simulink library "ADV_IP_MASTER"  (Simulink 8.6)
settings: Solver=VariableStepAuto  StartTime=0.0  StopTime=10.0  RelTol=1e-3
libraries: cdsEpicsOut x45, cdsFiltCtrl x25, cdsFilt x19, cdsEpicsIn x16, cdsTP x6, cdsMuxMatrix x4, VIS_LIB x1, cdsRampMuxMatrix x1, cdsFunctionCall x1, SIXOSEM_F_WD_AC_MASTER x1, SIXOSEM_F_STAGE_MASTER x1
(part 3 of 5)

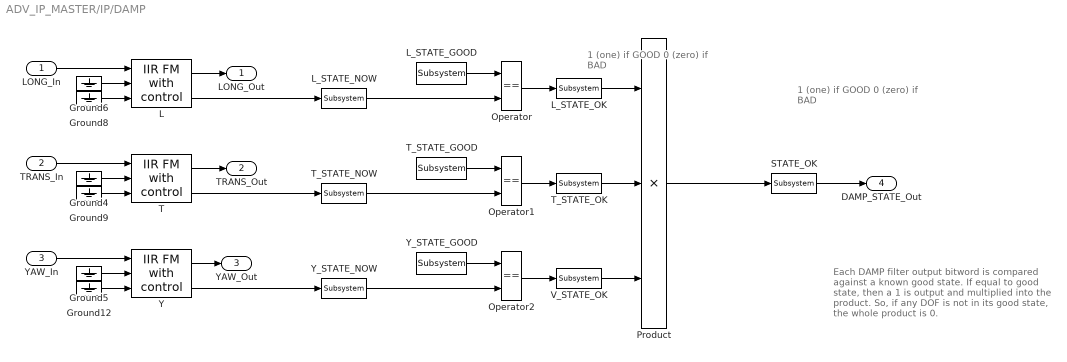
== system ADV_IP_MASTER/IP/DAMP ==
  note: 1 (one) if GOOD
      | 0 (zero) if BAD
  note: 1 (one) if GOOD
      | 0 (zero) if BAD
  note: Each DAMP filter output bitword is
      | compared against a known good state.
      | If equal to good state, then a 1 is output
      | and multiplied into the product. So, if any DOF
      | is not in its good state, the whole product is 0.
  LONG_In : Inport
  TRANS_In : Inport  Port=2
  YAW_In : Inport  Port=3
  Ground{4..6,8..9,12} (6 alike) : Ground
  L : cdsFiltCtrl/IIR FM with control  Tag=cdsFiltCtrl  Description=|
      | cdsFiltCntrl is the standard IIR filter module (exactly the same as cdsFilt) but with added control data output 'Ctrl'. Filter module digital signal output appears on the first output, which is called 'Val'. 'Ctrl' output has a bit pattern encoding the state of filter's on/off switches (FM1 through FM10). The bit values are:
      |                                                                                                                                                                                                                                                                                                                                       
      | module 	hex	dec                                                                                                                                                                                                                                                                                                                       
      | -----------------------                                                                                                                                                                                                                                                                                                               
      | FM1	0x20                    32                                                                                                                                                                                                                                                                                                        
      | FM2	0x80                     128                                                                                                                                                                                                                                                                                                      
      | FM3	0x200                   512                                                                                                                                                                                                                                                                                                       
      | FM4	0x800                   2048                                                                                                                                                                                                                                                                                                      
      | FM5	0x2000                 8192                                                                                                                                                                                                                                                                                                       
      | FM6	0x8000                 32768                                                                                                                                                                                                                                                                                                      
      | FM7	0x20000                131072                                                                                                                                                                                                                                                                                                     
      | FM8	0x80000                 524288                                                                                                                                                                                                                                                                                                    
      | FM9	0x200000               2097152                                                                                                                                                                                                                                                                                                    
      | FM10	0x800000               8388608                                                                                                                                                                                                                                                                                                   
      |                                                                                                                                                                                                                                                                                                                                       
      | This bit data can be used to drive some other switches or it can be output using a binary I/O module.
      settings: AttributesFormatString=%<Tag>
  L_STATE_GOOD : cdsEpicsIn/Subsystem  Tag=cdsEpicsIn  Description=|
      | Purpose:                                                                              
      | Create an EPICS input channel connection to the FE realtime controls.                 
      |                                                                                       
      | Operation:                                                                            
      | Outputs value from an EPICS ai record. Value is floating point with a precision of 3..
      |                                                                                       
      | Usage:                                                                                
      | Name the part with the desired EPICS channel name.
      settings: AttributesFormatString=%<Tag>
  L_STATE_NOW : cdsEpicsOut/Subsystem  Tag=cdsEpicsOutput  Description=|
      | Purpose:                                          
      | Output a FE signal to an EPICS channel.           
      |                                                   
      | Operation:                                        
      | Takes input value and passes it to EPICS record.  
      |                                                   
      | Usage:                                            
      | Name the part with the desired EPICS rrecord name.
      settings: AttributesFormatString=%<Tag>
  L_STATE_OK : cdsEpicsOut/Subsystem  Tag=cdsEpicsOutput  Description=|
      | Purpose:                                          
      | Output a FE signal to an EPICS channel.           
      |                                                   
      | Operation:                                        
      | Takes input value and passes it to EPICS record.  
      |                                                   
      | Usage:                                            
      | Name the part with the desired EPICS rrecord name.
      settings: AttributesFormatString=%<Tag>
  Operator : RelationalOperator  Operator===  OutDataTypeStr=boolean
  Operator1 : RelationalOperator  Operator===  OutDataTypeStr=boolean
  Operator2 : RelationalOperator  Operator===  OutDataTypeStr=boolean
  Product : Product  Inputs=3  RndMeth=Zero
  STATE_OK : cdsEpicsOut/Subsystem  Tag=cdsEpicsOutput  Description=|
      | Purpose:                                          
      | Output a FE signal to an EPICS channel.           
      |                                                   
      | Operation:                                        
      | Takes input value and passes it to EPICS record.  
      |                                                   
      | Usage:                                            
      | Name the part with the desired EPICS rrecord name.
      settings: AttributesFormatString=%<Tag>
  T : cdsFiltCtrl/IIR FM with control  Tag=cdsFiltCtrl  Description=|
      | cdsFiltCntrl is the standard IIR filter module (exactly the same as cdsFilt) but with added control data output 'Ctrl'. Filter module digital signal output appears on the first output, which is called 'Val'. 'Ctrl' output has a bit pattern encoding the state of filter's on/off switches (FM1 through FM10). The bit values are:
      |                                                                                                                                                                                                                                                                                                                                       
      | module 	hex	dec                                                                                                                                                                                                                                                                                                                       
      | -----------------------                                                                                                                                                                                                                                                                                                               
      | FM1	0x20                    32                                                                                                                                                                                                                                                                                                        
      | FM2	0x80                     128                                                                                                                                                                                                                                                                                                      
      | FM3	0x200                   512                                                                                                                                                                                                                                                                                                       
      | FM4	0x800                   2048                                                                                                                                                                                                                                                                                                      
      | FM5	0x2000                 8192                                                                                                                                                                                                                                                                                                       
      | FM6	0x8000                 32768                                                                                                                                                                                                                                                                                                      
      | FM7	0x20000                131072                                                                                                                                                                                                                                                                                                     
      | FM8	0x80000                 524288                                                                                                                                                                                                                                                                                                    
      | FM9	0x200000               2097152                                                                                                                                                                                                                                                                                                    
      | FM10	0x800000               8388608                                                                                                                                                                                                                                                                                                   
      |                                                                                                                                                                                                                                                                                                                                       
      | This bit data can be used to drive some other switches or it can be output using a binary I/O module.
      settings: AttributesFormatString=%<Tag>
  T_STATE_GOOD : cdsEpicsIn/Subsystem  Tag=cdsEpicsIn  Description=|
      | Purpose:                                                                              
      | Create an EPICS input channel connection to the FE realtime controls.                 
      |                                                                                       
      | Operation:                                                                            
      | Outputs value from an EPICS ai record. Value is floating point with a precision of 3..
      |                                                                                       
      | Usage:                                                                                
      | Name the part with the desired EPICS channel name.
      settings: AttributesFormatString=%<Tag>
  T_STATE_NOW : cdsEpicsOut/Subsystem  Tag=cdsEpicsOutput  Description=|
      | Purpose:                                          
      | Output a FE signal to an EPICS channel.           
      |                                                   
      | Operation:                                        
      | Takes input value and passes it to EPICS record.  
      |                                                   
      | Usage:                                            
      | Name the part with the desired EPICS rrecord name.
      settings: AttributesFormatString=%<Tag>
  T_STATE_OK : cdsEpicsOut/Subsystem  Tag=cdsEpicsOutput  Description=|
      | Purpose:                                          
      | Output a FE signal to an EPICS channel.           
      |                                                   
      | Operation:                                        
      | Takes input value and passes it to EPICS record.  
      |                                                   
      | Usage:                                            
      | Name the part with the desired EPICS rrecord name.
      settings: AttributesFormatString=%<Tag>
  V_STATE_OK : cdsEpicsOut/Subsystem  Tag=cdsEpicsOutput  Description=|
      | Purpose:                                          
      | Output a FE signal to an EPICS channel.           
      |                                                   
      | Operation:                                        
      | Takes input value and passes it to EPICS record.  
      |                                                   
      | Usage:                                            
      | Name the part with the desired EPICS rrecord name.
      settings: AttributesFormatString=%<Tag>
  Y : cdsFiltCtrl/IIR FM with control  Tag=cdsFiltCtrl  Description=|
      | cdsFiltCntrl is the standard IIR filter module (exactly the same as cdsFilt) but with added control data output 'Ctrl'. Filter module digital signal output appears on the first output, which is called 'Val'. 'Ctrl' output has a bit pattern encoding the state of filter's on/off switches (FM1 through FM10). The bit values are:
      |                                                                                                                                                                                                                                                                                                                                       
      | module 	hex	dec                                                                                                                                                                                                                                                                                                                       
      | -----------------------                                                                                                                                                                                                                                                                                                               
      | FM1	0x20                    32                                                                                                                                                                                                                                                                                                        
      | FM2	0x80                     128                                                                                                                                                                                                                                                                                                      
      | FM3	0x200                   512                                                                                                                                                                                                                                                                                                       
      | FM4	0x800                   2048                                                                                                                                                                                                                                                                                                      
      | FM5	0x2000                 8192                                                                                                                                                                                                                                                                                                       
      | FM6	0x8000                 32768                                                                                                                                                                                                                                                                                                      
      | FM7	0x20000                131072                                                                                                                                                                                                                                                                                                     
      | FM8	0x80000                 524288                                                                                                                                                                                                                                                                                                    
      | FM9	0x200000               2097152                                                                                                                                                                                                                                                                                                    
      | FM10	0x800000               8388608                                                                                                                                                                                                                                                                                                   
      |                                                                                                                                                                                                                                                                                                                                       
      | This bit data can be used to drive some other switches or it can be output using a binary I/O module.
      settings: AttributesFormatString=%<Tag>
  Y_STATE_GOOD : cdsEpicsIn/Subsystem  Tag=cdsEpicsIn  Description=|
      | Purpose:                                                                              
      | Create an EPICS input channel connection to the FE realtime controls.                 
      |                                                                                       
      | Operation:                                                                            
      | Outputs value from an EPICS ai record. Value is floating point with a precision of 3..
      |                                                                                       
      | Usage:                                                                                
      | Name the part with the desired EPICS channel name.
      settings: AttributesFormatString=%<Tag>
  Y_STATE_NOW : cdsEpicsOut/Subsystem  Tag=cdsEpicsOutput  Description=|
      | Purpose:                                          
      | Output a FE signal to an EPICS channel.           
      |                                                   
      | Operation:                                        
      | Takes input value and passes it to EPICS record.  
      |                                                   
      | Usage:                                            
      | Name the part with the desired EPICS rrecord name.
      settings: AttributesFormatString=%<Tag>
  LONG_Out : Outport
  TRANS_Out : Outport  Port=2
  YAW_Out : Outport  Port=3
  DAMP_STATE_Out : Outport  Port=4
  wires:
  Ground12/1 -> Y/3
  Ground9/1 -> T/3
  Ground8/1 -> L/3
  STATE_OK/1 -> DAMP_STATE_Out/1
  Y_STATE_NOW/1 -> Operator2/2
  T_STATE_NOW/1 -> Operator1/2
  L_STATE_NOW/1 -> Operator/2
  V_STATE_OK/1 -> Product/3
  T_STATE_OK/1 -> Product/2
  L_STATE_OK/1 -> Product/1
  Operator2/1 -> V_STATE_OK/1
  Operator1/1 -> T_STATE_OK/1
  Operator/1 -> L_STATE_OK/1
  Product/1 -> STATE_OK/1
  Y/2 -> Y_STATE_NOW/1
  Y_STATE_GOOD/1 -> Operator2/1
  T/2 -> T_STATE_NOW/1
  T_STATE_GOOD/1 -> Operator1/1
  L/2 -> L_STATE_NOW/1
  L_STATE_GOOD/1 -> Operator/1
  TRANS_In/1 -> T/1
  YAW_In/1 -> Y/1
  T/1 -> TRANS_Out/1
  Y/1 -> YAW_Out/1
  L/1 -> LONG_Out/1
  LONG_In/1 -> L/1
  Ground5/1 -> Y/2
  Ground4/1 -> T/2
  Ground6/1 -> L/2

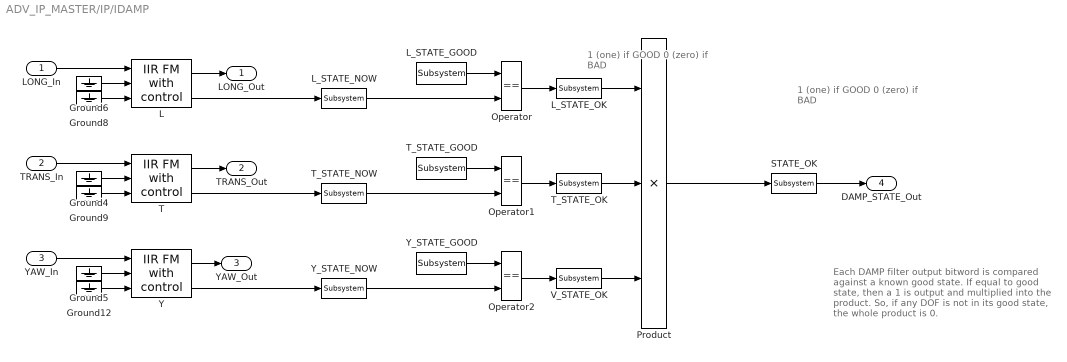
== system ADV_IP_MASTER/IP/IDAMP ==
  note: 1 (one) if GOOD
      | 0 (zero) if BAD
  note: 1 (one) if GOOD
      | 0 (zero) if BAD
  note: Each DAMP filter output bitword is
      | compared against a known good state.
      | If equal to good state, then a 1 is output
      | and multiplied into the product. So, if any DOF
      | is not in its good state, the whole product is 0.
  LONG_In : Inport
  TRANS_In : Inport  Port=2
  YAW_In : Inport  Port=3
  Ground{4..6,8..9,12} (6 alike) : Ground
  L : cdsFiltCtrl/IIR FM with control  Tag=cdsFiltCtrl  Description=|
      | cdsFiltCntrl is the standard IIR filter module (exactly the same as cdsFilt) but with added control data output 'Ctrl'. Filter module digital signal output appears on the first output, which is called 'Val'. 'Ctrl' output has a bit pattern encoding the state of filter's on/off switches (FM1 through FM10). The bit values are:
      |                                                                                                                                                                                                                                                                                                                                       
      | module 	hex	dec                                                                                                                                                                                                                                                                                                                       
      | -----------------------                                                                                                                                                                                                                                                                                                               
      | FM1	0x20                    32                                                                                                                                                                                                                                                                                                        
      | FM2	0x80                     128                                                                                                                                                                                                                                                                                                      
      | FM3	0x200                   512                                                                                                                                                                                                                                                                                                       
      | FM4	0x800                   2048                                                                                                                                                                                                                                                                                                      
      | FM5	0x2000                 8192                                                                                                                                                                                                                                                                                                       
      | FM6	0x8000                 32768                                                                                                                                                                                                                                                                                                      
      | FM7	0x20000                131072                                                                                                                                                                                                                                                                                                     
      | FM8	0x80000                 524288                                                                                                                                                                                                                                                                                                    
      | FM9	0x200000               2097152                                                                                                                                                                                                                                                                                                    
      | FM10	0x800000               8388608                                                                                                                                                                                                                                                                                                   
      |                                                                                                                                                                                                                                                                                                                                       
      | This bit data can be used to drive some other switches or it can be output using a binary I/O module.
      settings: AttributesFormatString=%<Tag>
  L_STATE_GOOD : cdsEpicsIn/Subsystem  Tag=cdsEpicsIn  Description=|
      | Purpose:                                                                              
      | Create an EPICS input channel connection to the FE realtime controls.                 
      |                                                                                       
      | Operation:                                                                            
      | Outputs value from an EPICS ai record. Value is floating point with a precision of 3..
      |                                                                                       
      | Usage:                                                                                
      | Name the part with the desired EPICS channel name.
      settings: AttributesFormatString=%<Tag>
  L_STATE_NOW : cdsEpicsOut/Subsystem  Tag=cdsEpicsOutput  Description=|
      | Purpose:                                          
      | Output a FE signal to an EPICS channel.           
      |                                                   
      | Operation:                                        
      | Takes input value and passes it to EPICS record.  
      |                                                   
      | Usage:                                            
      | Name the part with the desired EPICS rrecord name.
      settings: AttributesFormatString=%<Tag>
  L_STATE_OK : cdsEpicsOut/Subsystem  Tag=cdsEpicsOutput  Description=|
      | Purpose:                                          
      | Output a FE signal to an EPICS channel.           
      |                                                   
      | Operation:                                        
      | Takes input value and passes it to EPICS record.  
      |                                                   
      | Usage:                                            
      | Name the part with the desired EPICS rrecord name.
      settings: AttributesFormatString=%<Tag>
  Operator : RelationalOperator  Operator===  OutDataTypeStr=boolean
  Operator1 : RelationalOperator  Operator===  OutDataTypeStr=boolean
  Operator2 : RelationalOperator  Operator===  OutDataTypeStr=boolean
  Product : Product  Inputs=3  RndMeth=Zero
  STATE_OK : cdsEpicsOut/Subsystem  Tag=cdsEpicsOutput  Description=|
      | Purpose:                                          
      | Output a FE signal to an EPICS channel.           
      |                                                   
      | Operation:                                        
      | Takes input value and passes it to EPICS record.  
      |                                                   
      | Usage:                                            
      | Name the part with the desired EPICS rrecord name.
      settings: AttributesFormatString=%<Tag>
  T : cdsFiltCtrl/IIR FM with control  Tag=cdsFiltCtrl  Description=|
      | cdsFiltCntrl is the standard IIR filter module (exactly the same as cdsFilt) but with added control data output 'Ctrl'. Filter module digital signal output appears on the first output, which is called 'Val'. 'Ctrl' output has a bit pattern encoding the state of filter's on/off switches (FM1 through FM10). The bit values are:
      |                                                                                                                                                                                                                                                                                                                                       
      | module 	hex	dec                                                                                                                                                                                                                                                                                                                       
      | -----------------------                                                                                                                                                                                                                                                                                                               
      | FM1	0x20                    32                                                                                                                                                                                                                                                                                                        
      | FM2	0x80                     128                                                                                                                                                                                                                                                                                                      
      | FM3	0x200                   512                                                                                                                                                                                                                                                                                                       
      | FM4	0x800                   2048                                                                                                                                                                                                                                                                                                      
      | FM5	0x2000                 8192                                                                                                                                                                                                                                                                                                       
      | FM6	0x8000                 32768                                                                                                                                                                                                                                                                                                      
      | FM7	0x20000                131072                                                                                                                                                                                                                                                                                                     
      | FM8	0x80000                 524288                                                                                                                                                                                                                                                                                                    
      | FM9	0x200000               2097152                                                                                                                                                                                                                                                                                                    
      | FM10	0x800000               8388608                                                                                                                                                                                                                                                                                                   
      |                                                                                                                                                                                                                                                                                                                                       
      | This bit data can be used to drive some other switches or it can be output using a binary I/O module.
      settings: AttributesFormatString=%<Tag>
  T_STATE_GOOD : cdsEpicsIn/Subsystem  Tag=cdsEpicsIn  Description=|
      | Purpose:                                                                              
      | Create an EPICS input channel connection to the FE realtime controls.                 
      |                                                                                       
      | Operation:                                                                            
      | Outputs value from an EPICS ai record. Value is floating point with a precision of 3..
      |                                                                                       
      | Usage:                                                                                
      | Name the part with the desired EPICS channel name.
      settings: AttributesFormatString=%<Tag>
  T_STATE_NOW : cdsEpicsOut/Subsystem  Tag=cdsEpicsOutput  Description=|
      | Purpose:                                          
      | Output a FE signal to an EPICS channel.           
      |                                                   
      | Operation:                                        
      | Takes input value and passes it to EPICS record.  
      |                                                   
      | Usage:                                            
      | Name the part with the desired EPICS rrecord name.
      settings: AttributesFormatString=%<Tag>
  T_STATE_OK : cdsEpicsOut/Subsystem  Tag=cdsEpicsOutput  Description=|
      | Purpose:                                          
      | Output a FE signal to an EPICS channel.           
      |                                                   
      | Operation:                                        
      | Takes input value and passes it to EPICS record.  
      |                                                   
      | Usage:                                            
      | Name the part with the desired EPICS rrecord name.
      settings: AttributesFormatString=%<Tag>
  V_STATE_OK : cdsEpicsOut/Subsystem  Tag=cdsEpicsOutput  Description=|
      | Purpose:                                          
      | Output a FE signal to an EPICS channel.           
      |                                                   
      | Operation:                                        
      | Takes input value and passes it to EPICS record.  
      |                                                   
      | Usage:                                            
      | Name the part with the desired EPICS rrecord name.
      settings: AttributesFormatString=%<Tag>
  Y : cdsFiltCtrl/IIR FM with control  Tag=cdsFiltCtrl  Description=|
      | cdsFiltCntrl is the standard IIR filter module (exactly the same as cdsFilt) but with added control data output 'Ctrl'. Filter module digital signal output appears on the first output, which is called 'Val'. 'Ctrl' output has a bit pattern encoding the state of filter's on/off switches (FM1 through FM10). The bit values are:
      |                                                                                                                                                                                                                                                                                                                                       
      | module 	hex	dec                                                                                                                                                                                                                                                                                                                       
      | -----------------------                                                                                                                                                                                                                                                                                                               
      | FM1	0x20                    32                                                                                                                                                                                                                                                                                                        
      | FM2	0x80                     128                                                                                                                                                                                                                                                                                                      
      | FM3	0x200                   512                                                                                                                                                                                                                                                                                                       
      | FM4	0x800                   2048                                                                                                                                                                                                                                                                                                      
      | FM5	0x2000                 8192                                                                                                                                                                                                                                                                                                       
      | FM6	0x8000                 32768                                                                                                                                                                                                                                                                                                      
      | FM7	0x20000                131072                                                                                                                                                                                                                                                                                                     
      | FM8	0x80000                 524288                                                                                                                                                                                                                                                                                                    
      | FM9	0x200000               2097152                                                                                                                                                                                                                                                                                                    
      | FM10	0x800000               8388608                                                                                                                                                                                                                                                                                                   
      |                                                                                                                                                                                                                                                                                                                                       
      | This bit data can be used to drive some other switches or it can be output using a binary I/O module.
      settings: AttributesFormatString=%<Tag>
  Y_STATE_GOOD : cdsEpicsIn/Subsystem  Tag=cdsEpicsIn  Description=|
      | Purpose:                                                                              
      | Create an EPICS input channel connection to the FE realtime controls.                 
      |                                                                                       
      | Operation:                                                                            
      | Outputs value from an EPICS ai record. Value is floating point with a precision of 3..
      |                                                                                       
      | Usage:                                                                                
      | Name the part with the desired EPICS channel name.
      settings: AttributesFormatString=%<Tag>
  Y_STATE_NOW : cdsEpicsOut/Subsystem  Tag=cdsEpicsOutput  Description=|
      | Purpose:                                          
      | Output a FE signal to an EPICS channel.           
      |                                                   
      | Operation:                                        
      | Takes input value and passes it to EPICS record.  
      |                                                   
      | Usage:                                            
      | Name the part with the desired EPICS rrecord name.
      settings: AttributesFormatString=%<Tag>
  LONG_Out : Outport
  TRANS_Out : Outport  Port=2
  YAW_Out : Outport  Port=3
  DAMP_STATE_Out : Outport  Port=4
  wires:
  Ground12/1 -> Y/3
  Ground9/1 -> T/3
  Ground8/1 -> L/3
  STATE_OK/1 -> DAMP_STATE_Out/1
  Y_STATE_NOW/1 -> Operator2/2
  T_STATE_NOW/1 -> Operator1/2
  L_STATE_NOW/1 -> Operator/2
  V_STATE_OK/1 -> Product/3
  T_STATE_OK/1 -> Product/2
  L_STATE_OK/1 -> Product/1
  Operator2/1 -> V_STATE_OK/1
  Operator1/1 -> T_STATE_OK/1
  Operator/1 -> L_STATE_OK/1
  Product/1 -> STATE_OK/1
  Y/2 -> Y_STATE_NOW/1
  Y_STATE_GOOD/1 -> Operator2/1
  T/2 -> T_STATE_NOW/1
  T_STATE_GOOD/1 -> Operator1/1
  L/2 -> L_STATE_NOW/1
  L_STATE_GOOD/1 -> Operator/1
  TRANS_In/1 -> T/1
  YAW_In/1 -> Y/1
  T/1 -> TRANS_Out/1
  Y/1 -> YAW_Out/1
  L/1 -> LONG_Out/1
  LONG_In/1 -> L/1
  Ground5/1 -> Y/2
  Ground4/1 -> T/2
  Ground6/1 -> L/2
